simulink model "simple_router"  (R2015a)
settings: Solver=ode45  StartTime=0.0  StopTime=3000  FixedStep=1  RelTol=1e-3
undefined symbols (not defined in the file or in its folder): des, SELECT, T
libraries: simulink x16
(part 4 of 6)

== system simple_router/PE3/Create Generator Selection Variable ==
  function : TriggerPort  TriggerType=function-call
  Repeating Sequence Stair : simulink/Sources/Repeating Sequence Stair  OutValues=[0 1].'  tsamp=-1  OutMin=[]  OutMax=[]  OutDataTypeStr=float('double')  OutputDataTypeScalingMode=Specify via dialog  OutDataType=float('double')  ConRadixGroup=Best Precision: Vector-wise  OutScaling=2^-12
  Out1 : Outport
  wires:
  Repeating Sequence Stair/1 -> Out1/1

== system simple_router/PE4/Create Generator Selection Variable ==
  function : TriggerPort  TriggerType=function-call
  Repeating Sequence Stair : simulink/Sources/Repeating Sequence Stair  OutValues=[0 1].'  tsamp=-1  OutMin=[]  OutMax=[]  OutDataTypeStr=float('double')  OutputDataTypeScalingMode=Specify via dialog  OutDataType=float('double')  ConRadixGroup=Best Precision: Vector-wise  OutScaling=2^-12
  Out1 : Outport
  wires:
  Repeating Sequence Stair/1 -> Out1/1

== system simple_router/PE5/Create Generator Selection Variable ==
  function : TriggerPort  TriggerType=function-call
  Repeating Sequence Stair : simulink/Sources/Repeating Sequence Stair  OutValues=[0 1].'  tsamp=-1  OutMin=[]  OutMax=[]  OutDataTypeStr=float('double')  OutputDataTypeScalingMode=Specify via dialog  OutDataType=float('double')  ConRadixGroup=Best Precision: Vector-wise  OutScaling=2^-12
  Out1 : Outport
  wires:
  Repeating Sequence Stair/1 -> Out1/1

== system simple_router/PE6/Create Generator Selection Variable ==
  function : TriggerPort  TriggerType=function-call
  Repeating Sequence Stair : simulink/Sources/Repeating Sequence Stair  OutValues=[0 1].'  tsamp=-1  OutMin=[]  OutMax=[]  OutDataTypeStr=float('double')  OutputDataTypeScalingMode=Specify via dialog  OutDataType=float('double')  ConRadixGroup=Best Precision: Vector-wise  OutScaling=2^-12
  Out1 : Outport
  wires:
  Repeating Sequence Stair/1 -> Out1/1

== system simple_router/PE7/Create Generator Selection Variable ==
  function : TriggerPort  TriggerType=function-call
  Repeating Sequence Stair : simulink/Sources/Repeating Sequence Stair  OutValues=[0 1].'  tsamp=-1  OutMin=[]  OutMax=[]  OutDataTypeStr=float('double')  OutputDataTypeScalingMode=Specify via dialog  OutDataType=float('double')  ConRadixGroup=Best Precision: Vector-wise  OutScaling=2^-12
  Out1 : Outport
  wires:
  Repeating Sequence Stair/1 -> Out1/1

== system simple_router/PE8/Create Generator Selection Variable ==
  function : TriggerPort  TriggerType=function-call
  Repeating Sequence Stair : simulink/Sources/Repeating Sequence Stair  OutValues=[0 1].'  tsamp=-1  OutMin=[]  OutMax=[]  OutDataTypeStr=float('double')  OutputDataTypeScalingMode=Specify via dialog  OutDataType=float('double')  ConRadixGroup=Best Precision: Vector-wise  OutScaling=2^-12
  Out1 : Outport
  wires:
  Repeating Sequence Stair/1 -> Out1/1

== system simple_router/PE9/Create Generator Selection Variable ==
  function : TriggerPort  TriggerType=function-call
  Repeating Sequence Stair : simulink/Sources/Repeating Sequence Stair  OutValues=[0 1].'  tsamp=-1  OutMin=[]  OutMax=[]  OutDataTypeStr=float('double')  OutputDataTypeScalingMode=Specify via dialog  OutDataType=float('double')  ConRadixGroup=Best Precision: Vector-wise  OutScaling=2^-12
  Out1 : Outport
  wires:
  Repeating Sequence Stair/1 -> Out1/1

== system simple_router/Router00/Attribute Function ==
  MATLAB Function : MATLAB Function  TreatAsAtomicUnit=on
  __DMLF__EDE2FCE__ : EntityDepartureFunctionCallGenerator  TimingFunctionCallF1=Before entity departure  IsInsideAFB=on
  __DMLF__GA__ : GetAttribute  AttributeName=DST|ME  AttributeMissing=Error|Error  AttributeDefaultValue=1|1  AttributeTreatAsVector=1|1  AttributeSendTiming=Before entity departure|Before entity departure  EvaluatedDefaultAttributeValue={ [];[]}  IsInsideAFB=on
      settings: OutputPortMap=o1,o2
  __DMLF__SA__ : SetAttribute  AttributeName=RT  AttributeFrom=Signal port  EvaluatedAttributeValue={ []}  IsInsideAFB=on
  IN : PMIOPort  Port=1  Side=Left
  OUT : PMIOPort  Port=2  Side=Right
  wires:
  __DMLF__EDE2FCE__/1 -> MATLAB Function/Trigger
  __DMLF__GA__/1 -> MATLAB Function/1(DST)
  __DMLF__GA__/2 -> MATLAB Function/2(ME)
  MATLAB Function/1(out_RT) -> __DMLF__SA__/1
  connections:
  __DMLF__SA__/LConn1 -- __DMLF__EDE2FCE__/RConn1
  __DMLF__GA__/RConn1 -- __DMLF__EDE2FCE__/LConn1
  IN/RConn1 -- __DMLF__GA__/LConn1
  __DMLF__SA__/RConn1 -- OUT/RConn1

== system simple_router/Router00/Clocked FIFO1 ==
  Event-Based Random Number : EventBasedRandomNumber  Distribution=Gaussian (normal)  meanNorm=E  stdNorm=S
  FIFO Queue : FIFOQueue  Capacity=F  StatNumberInBlock=on
      settings: OutputPortMap=o1
  Release Gate : ReleaseGate  OpenGateUpon=Function call from port fcn
  Time-Based Function-Call Generator : TimeBasedFunctionCallGenerator  EventGenerationMode=Period from port  Period=T
  Input : PMIOPort  Port=1  Side=Left
  Output : PMIOPort  Port=2  Side=Right
  #n : Outport
  wires:
  Time-Based Function-Call Generator/1 -> Release Gate/1
  FIFO Queue/1 -> #n/1
  Event-Based Random Number/1 -> Time-Based Function-Call Generator/1
  connections:
  FIFO Queue/LConn1 -- Input/RConn1
  Release Gate/RConn1 -- Output/RConn1
  FIFO Queue/RConn1 -- Release Gate/LConn1

== system simple_router/Router00/Clocked FIFO2 ==
  Event-Based Random Number : EventBasedRandomNumber  Distribution=Gaussian (normal)  meanNorm=E  stdNorm=S
  FIFO Queue : FIFOQueue  Capacity=F  StatNumberInBlock=on
      settings: OutputPortMap=o1
  Release Gate : ReleaseGate  OpenGateUpon=Function call from port fcn
  Time-Based Function-Call Generator : TimeBasedFunctionCallGenerator  EventGenerationMode=Period from port  Period=T
  Input : PMIOPort  Port=1  Side=Left
  Output : PMIOPort  Port=2  Side=Right
  #n : Outport
  wires:
  Time-Based Function-Call Generator/1 -> Release Gate/1
  FIFO Queue/1 -> #n/1
  Event-Based Random Number/1 -> Time-Based Function-Call Generator/1
  connections:
  FIFO Queue/LConn1 -- Input/RConn1
  Release Gate/RConn1 -- Output/RConn1
  FIFO Queue/RConn1 -- Release Gate/LConn1

== system simple_router/Router00/Clocked FIFO3 ==
  Event-Based Random Number : EventBasedRandomNumber  Distribution=Gaussian (normal)  meanNorm=E  stdNorm=S
  FIFO Queue : FIFOQueue  Capacity=F  StatNumberInBlock=on
      settings: OutputPortMap=o1
  Release Gate : ReleaseGate  OpenGateUpon=Function call from port fcn
  Time-Based Function-Call Generator : TimeBasedFunctionCallGenerator  EventGenerationMode=Period from port  Period=T
  Input : PMIOPort  Port=1  Side=Left
  Output : PMIOPort  Port=2  Side=Right
  #n : Outport
  wires:
  Time-Based Function-Call Generator/1 -> Release Gate/1
  FIFO Queue/1 -> #n/1
  Event-Based Random Number/1 -> Time-Based Function-Call Generator/1
  connections:
  FIFO Queue/LConn1 -- Input/RConn1
  Release Gate/RConn1 -- Output/RConn1
  FIFO Queue/RConn1 -- Release Gate/LConn1

== system simple_router/Router00/Clocked FIFO4 ==
  Event-Based Random Number : EventBasedRandomNumber  Distribution=Gaussian (normal)  meanNorm=E  stdNorm=S
  FIFO Queue : FIFOQueue  Capacity=F  StatNumberInBlock=on
      settings: OutputPortMap=o1
  Release Gate : ReleaseGate  OpenGateUpon=Function call from port fcn
  Time-Based Function-Call Generator : TimeBasedFunctionCallGenerator  EventGenerationMode=Period from port  Period=T
  Input : PMIOPort  Port=1  Side=Left
  Output : PMIOPort  Port=2  Side=Right
  #n : Outport
  wires:
  Time-Based Function-Call Generator/1 -> Release Gate/1
  FIFO Queue/1 -> #n/1
  Event-Based Random Number/1 -> Time-Based Function-Call Generator/1
  connections:
  FIFO Queue/LConn1 -- Input/RConn1
  Release Gate/RConn1 -- Output/RConn1
  FIFO Queue/RConn1 -- Release Gate/LConn1

== system simple_router/Router00/Clocked FIFO5 ==
  Event-Based Random Number : EventBasedRandomNumber  Distribution=Gaussian (normal)  meanNorm=E  stdNorm=S
  FIFO Queue : FIFOQueue  Capacity=F  StatNumberInBlock=on
      settings: OutputPortMap=o1
  Release Gate : ReleaseGate  OpenGateUpon=Function call from port fcn
  Time-Based Function-Call Generator : TimeBasedFunctionCallGenerator  EventGenerationMode=Period from port  Period=T
  Input : PMIOPort  Port=1  Side=Left
  Output : PMIOPort  Port=2  Side=Right
  #n : Outport
  wires:
  Time-Based Function-Call Generator/1 -> Release Gate/1
  FIFO Queue/1 -> #n/1
  Event-Based Random Number/1 -> Time-Based Function-Call Generator/1
  connections:
  FIFO Queue/LConn1 -- Input/RConn1
  Release Gate/RConn1 -- Output/RConn1
  FIFO Queue/RConn1 -- Release Gate/LConn1

== system simple_router/Router01/Attribute Function ==
  MATLAB Function : MATLAB Function  TreatAsAtomicUnit=on
  __DMLF__EDE2FCE__ : EntityDepartureFunctionCallGenerator  TimingFunctionCallF1=Before entity departure  IsInsideAFB=on
  __DMLF__GA__ : GetAttribute  AttributeName=DST|ME  AttributeMissing=Error|Error  AttributeDefaultValue=1|1  AttributeTreatAsVector=1|1  AttributeSendTiming=Before entity departure|Before entity departure  EvaluatedDefaultAttributeValue={ [];[]}  IsInsideAFB=on
      settings: OutputPortMap=o1,o2
  __DMLF__SA__ : SetAttribute  AttributeName=RT  AttributeFrom=Signal port  EvaluatedAttributeValue={ []}  IsInsideAFB=on
  IN : PMIOPort  Port=1  Side=Left
  OUT : PMIOPort  Port=2  Side=Right
  wires:
  __DMLF__EDE2FCE__/1 -> MATLAB Function/Trigger
  __DMLF__GA__/1 -> MATLAB Function/1(DST)
  __DMLF__GA__/2 -> MATLAB Function/2(ME)
  MATLAB Function/1(out_RT) -> __DMLF__SA__/1
  connections:
  __DMLF__SA__/LConn1 -- __DMLF__EDE2FCE__/RConn1
  __DMLF__GA__/RConn1 -- __DMLF__EDE2FCE__/LConn1
  IN/RConn1 -- __DMLF__GA__/LConn1
  __DMLF__SA__/RConn1 -- OUT/RConn1

== system simple_router/Router01/Clocked FIFO1 ==
  Event-Based Random Number : EventBasedRandomNumber  Distribution=Gaussian (normal)  meanNorm=E  stdNorm=S
  FIFO Queue : FIFOQueue  Capacity=F  StatNumberInBlock=on
      settings: OutputPortMap=o1
  Release Gate : ReleaseGate  OpenGateUpon=Function call from port fcn
  Time-Based Function-Call Generator : TimeBasedFunctionCallGenerator  EventGenerationMode=Period from port  Period=T
  Input : PMIOPort  Port=1  Side=Left
  Output : PMIOPort  Port=2  Side=Right
  #n : Outport
  wires:
  Time-Based Function-Call Generator/1 -> Release Gate/1
  FIFO Queue/1 -> #n/1
  Event-Based Random Number/1 -> Time-Based Function-Call Generator/1
  connections:
  FIFO Queue/LConn1 -- Input/RConn1
  Release Gate/RConn1 -- Output/RConn1
  FIFO Queue/RConn1 -- Release Gate/LConn1

== system simple_router/Router01/Clocked FIFO2 ==
  Event-Based Random Number : EventBasedRandomNumber  Distribution=Gaussian (normal)  meanNorm=E  stdNorm=S
  FIFO Queue : FIFOQueue  Capacity=F  StatNumberInBlock=on
      settings: OutputPortMap=o1
  Release Gate : ReleaseGate  OpenGateUpon=Function call from port fcn
  Time-Based Function-Call Generator : TimeBasedFunctionCallGenerator  EventGenerationMode=Period from port  Period=T
  Input : PMIOPort  Port=1  Side=Left
  Output : PMIOPort  Port=2  Side=Right
  #n : Outport
  wires:
  Time-Based Function-Call Generator/1 -> Release Gate/1
  FIFO Queue/1 -> #n/1
  Event-Based Random Number/1 -> Time-Based Function-Call Generator/1
  connections:
  FIFO Queue/LConn1 -- Input/RConn1
  Release Gate/RConn1 -- Output/RConn1
  FIFO Queue/RConn1 -- Release Gate/LConn1

== system simple_router/Router01/Clocked FIFO3 ==
  Event-Based Random Number : EventBasedRandomNumber  Distribution=Gaussian (normal)  meanNorm=E  stdNorm=S
  FIFO Queue : FIFOQueue  Capacity=F  StatNumberInBlock=on
      settings: OutputPortMap=o1
  Release Gate : ReleaseGate  OpenGateUpon=Function call from port fcn
  Time-Based Function-Call Generator : TimeBasedFunctionCallGenerator  EventGenerationMode=Period from port  Period=T
  Input : PMIOPort  Port=1  Side=Left
  Output : PMIOPort  Port=2  Side=Right
  #n : Outport
  wires:
  Time-Based Function-Call Generator/1 -> Release Gate/1
  FIFO Queue/1 -> #n/1
  Event-Based Random Number/1 -> Time-Based Function-Call Generator/1
  connections:
  FIFO Queue/LConn1 -- Input/RConn1
  Release Gate/RConn1 -- Output/RConn1
  FIFO Queue/RConn1 -- Release Gate/LConn1

== system simple_router/Router01/Clocked FIFO4 ==
  Event-Based Random Number : EventBasedRandomNumber  Distribution=Gaussian (normal)  meanNorm=E  stdNorm=S
  FIFO Queue : FIFOQueue  Capacity=F  StatNumberInBlock=on
      settings: OutputPortMap=o1
  Release Gate : ReleaseGate  OpenGateUpon=Function call from port fcn
  Time-Based Function-Call Generator : TimeBasedFunctionCallGenerator  EventGenerationMode=Period from port  Period=T
  Input : PMIOPort  Port=1  Side=Left
  Output : PMIOPort  Port=2  Side=Right
  #n : Outport
  wires:
  Time-Based Function-Call Generator/1 -> Release Gate/1
  FIFO Queue/1 -> #n/1
  Event-Based Random Number/1 -> Time-Based Function-Call Generator/1
  connections:
  FIFO Queue/LConn1 -- Input/RConn1
  Release Gate/RConn1 -- Output/RConn1
  FIFO Queue/RConn1 -- Release Gate/LConn1

== system simple_router/Router01/Clocked FIFO5 ==
  Event-Based Random Number : EventBasedRandomNumber  Distribution=Gaussian (normal)  meanNorm=E  stdNorm=S
  FIFO Queue : FIFOQueue  Capacity=F  StatNumberInBlock=on
      settings: OutputPortMap=o1
  Release Gate : ReleaseGate  OpenGateUpon=Function call from port fcn
  Time-Based Function-Call Generator : TimeBasedFunctionCallGenerator  EventGenerationMode=Period from port  Period=T
  Input : PMIOPort  Port=1  Side=Left
  Output : PMIOPort  Port=2  Side=Right
  #n : Outport
  wires:
  Time-Based Function-Call Generator/1 -> Release Gate/1
  FIFO Queue/1 -> #n/1
  Event-Based Random Number/1 -> Time-Based Function-Call Generator/1
  connections:
  FIFO Queue/LConn1 -- Input/RConn1
  Release Gate/RConn1 -- Output/RConn1
  FIFO Queue/RConn1 -- Release Gate/LConn1

== system simple_router/Router02/Attribute Function ==
  MATLAB Function : MATLAB Function  TreatAsAtomicUnit=on
  __DMLF__EDE2FCE__ : EntityDepartureFunctionCallGenerator  TimingFunctionCallF1=Before entity departure  IsInsideAFB=on
  __DMLF__GA__ : GetAttribute  AttributeName=DST|ME  AttributeMissing=Error|Error  AttributeDefaultValue=1|1  AttributeTreatAsVector=1|1  AttributeSendTiming=Before entity departure|Before entity departure  EvaluatedDefaultAttributeValue={ [];[]}  IsInsideAFB=on
      settings: OutputPortMap=o1,o2
  __DMLF__SA__ : SetAttribute  AttributeName=RT  AttributeFrom=Signal port  EvaluatedAttributeValue={ []}  IsInsideAFB=on
  IN : PMIOPort  Port=1  Side=Left
  OUT : PMIOPort  Port=2  Side=Right
  wires:
  __DMLF__EDE2FCE__/1 -> MATLAB Function/Trigger
  __DMLF__GA__/1 -> MATLAB Function/1(DST)
  __DMLF__GA__/2 -> MATLAB Function/2(ME)
  MATLAB Function/1(out_RT) -> __DMLF__SA__/1
  connections:
  __DMLF__SA__/LConn1 -- __DMLF__EDE2FCE__/RConn1
  __DMLF__GA__/RConn1 -- __DMLF__EDE2FCE__/LConn1
  IN/RConn1 -- __DMLF__GA__/LConn1
  __DMLF__SA__/RConn1 -- OUT/RConn1

== system simple_router/Router02/Clocked FIFO1 ==
  Event-Based Random Number : EventBasedRandomNumber  Distribution=Gaussian (normal)  meanNorm=E  stdNorm=S
  FIFO Queue : FIFOQueue  Capacity=F  StatNumberInBlock=on
      settings: OutputPortMap=o1
  Release Gate : ReleaseGate  OpenGateUpon=Function call from port fcn
  Time-Based Function-Call Generator : TimeBasedFunctionCallGenerator  EventGenerationMode=Period from port  Period=T
  Input : PMIOPort  Port=1  Side=Left
  Output : PMIOPort  Port=2  Side=Right
  #n : Outport
  wires:
  Time-Based Function-Call Generator/1 -> Release Gate/1
  FIFO Queue/1 -> #n/1
  Event-Based Random Number/1 -> Time-Based Function-Call Generator/1
  connections:
  FIFO Queue/LConn1 -- Input/RConn1
  Release Gate/RConn1 -- Output/RConn1
  FIFO Queue/RConn1 -- Release Gate/LConn1

== system simple_router/Router02/Clocked FIFO2 ==
  Event-Based Random Number : EventBasedRandomNumber  Distribution=Gaussian (normal)  meanNorm=E  stdNorm=S
  FIFO Queue : FIFOQueue  Capacity=F  StatNumberInBlock=on
      settings: OutputPortMap=o1
  Release Gate : ReleaseGate  OpenGateUpon=Function call from port fcn
  Time-Based Function-Call Generator : TimeBasedFunctionCallGenerator  EventGenerationMode=Period from port  Period=T
  Input : PMIOPort  Port=1  Side=Left
  Output : PMIOPort  Port=2  Side=Right
  #n : Outport
  wires:
  Time-Based Function-Call Generator/1 -> Release Gate/1
  FIFO Queue/1 -> #n/1
  Event-Based Random Number/1 -> Time-Based Function-Call Generator/1
  connections:
  FIFO Queue/LConn1 -- Input/RConn1
  Release Gate/RConn1 -- Output/RConn1
  FIFO Queue/RConn1 -- Release Gate/LConn1

== system simple_router/Router02/Clocked FIFO3 ==
  Event-Based Random Number : EventBasedRandomNumber  Distribution=Gaussian (normal)  meanNorm=E  stdNorm=S
  FIFO Queue : FIFOQueue  Capacity=F  StatNumberInBlock=on
      settings: OutputPortMap=o1
  Release Gate : ReleaseGate  OpenGateUpon=Function call from port fcn
  Time-Based Function-Call Generator : TimeBasedFunctionCallGenerator  EventGenerationMode=Period from port  Period=T
  Input : PMIOPort  Port=1  Side=Left
  Output : PMIOPort  Port=2  Side=Right
  #n : Outport
  wires:
  Time-Based Function-Call Generator/1 -> Release Gate/1
  FIFO Queue/1 -> #n/1
  Event-Based Random Number/1 -> Time-Based Function-Call Generator/1
  connections:
  FIFO Queue/LConn1 -- Input/RConn1
  Release Gate/RConn1 -- Output/RConn1
  FIFO Queue/RConn1 -- Release Gate/LConn1

== system simple_router/Router02/Clocked FIFO4 ==
  Event-Based Random Number : EventBasedRandomNumber  Distribution=Gaussian (normal)  meanNorm=E  stdNorm=S
  FIFO Queue : FIFOQueue  Capacity=F  StatNumberInBlock=on
      settings: OutputPortMap=o1
  Release Gate : ReleaseGate  OpenGateUpon=Function call from port fcn
  Time-Based Function-Call Generator : TimeBasedFunctionCallGenerator  EventGenerationMode=Period from port  Period=T
  Input : PMIOPort  Port=1  Side=Left
  Output : PMIOPort  Port=2  Side=Right
  #n : Outport
  wires:
  Time-Based Function-Call Generator/1 -> Release Gate/1
  FIFO Queue/1 -> #n/1
  Event-Based Random Number/1 -> Time-Based Function-Call Generator/1
  connections:
  FIFO Queue/LConn1 -- Input/RConn1
  Release Gate/RConn1 -- Output/RConn1
  FIFO Queue/RConn1 -- Release Gate/LConn1

== system simple_router/Router02/Clocked FIFO5 ==
  Event-Based Random Number : EventBasedRandomNumber  Distribution=Gaussian (normal)  meanNorm=E  stdNorm=S
  FIFO Queue : FIFOQueue  Capacity=F  StatNumberInBlock=on
      settings: OutputPortMap=o1
  Release Gate : ReleaseGate  OpenGateUpon=Function call from port fcn
  Time-Based Function-Call Generator : TimeBasedFunctionCallGenerator  EventGenerationMode=Period from port  Period=T
  Input : PMIOPort  Port=1  Side=Left
  Output : PMIOPort  Port=2  Side=Right
  #n : Outport
  wires:
  Time-Based Function-Call Generator/1 -> Release Gate/1
  FIFO Queue/1 -> #n/1
  Event-Based Random Number/1 -> Time-Based Function-Call Generator/1
  connections:
  FIFO Queue/LConn1 -- Input/RConn1
  Release Gate/RConn1 -- Output/RConn1
  FIFO Queue/RConn1 -- Release Gate/LConn1

== system simple_router/Router03/Attribute Function ==
  MATLAB Function : MATLAB Function  TreatAsAtomicUnit=on
  __DMLF__EDE2FCE__ : EntityDepartureFunctionCallGenerator  TimingFunctionCallF1=Before entity departure  IsInsideAFB=on
  __DMLF__GA__ : GetAttribute  AttributeName=DST|ME  AttributeMissing=Error|Error  AttributeDefaultValue=1|1  AttributeTreatAsVector=1|1  AttributeSendTiming=Before entity departure|Before entity departure  EvaluatedDefaultAttributeValue={ [];[]}  IsInsideAFB=on
      settings: OutputPortMap=o1,o2
  __DMLF__SA__ : SetAttribute  AttributeName=RT  AttributeFrom=Signal port  EvaluatedAttributeValue={ []}  IsInsideAFB=on
  IN : PMIOPort  Port=1  Side=Left
  OUT : PMIOPort  Port=2  Side=Right
  wires:
  __DMLF__EDE2FCE__/1 -> MATLAB Function/Trigger
  __DMLF__GA__/1 -> MATLAB Function/1(DST)
  __DMLF__GA__/2 -> MATLAB Function/2(ME)
  MATLAB Function/1(out_RT) -> __DMLF__SA__/1
  connections:
  __DMLF__SA__/LConn1 -- __DMLF__EDE2FCE__/RConn1
  __DMLF__GA__/RConn1 -- __DMLF__EDE2FCE__/LConn1
  IN/RConn1 -- __DMLF__GA__/LConn1
  __DMLF__SA__/RConn1 -- OUT/RConn1

== system simple_router/Router03/Clocked FIFO1 ==
  Event-Based Random Number : EventBasedRandomNumber  Distribution=Gaussian (normal)  meanNorm=E  stdNorm=S
  FIFO Queue : FIFOQueue  Capacity=F  StatNumberInBlock=on
      settings: OutputPortMap=o1
  Release Gate : ReleaseGate  OpenGateUpon=Function call from port fcn
  Time-Based Function-Call Generator : TimeBasedFunctionCallGenerator  EventGenerationMode=Period from port  Period=T
  Input : PMIOPort  Port=1  Side=Left
  Output : PMIOPort  Port=2  Side=Right
  #n : Outport
  wires:
  Time-Based Function-Call Generator/1 -> Release Gate/1
  FIFO Queue/1 -> #n/1
  Event-Based Random Number/1 -> Time-Based Function-Call Generator/1
  connections:
  FIFO Queue/LConn1 -- Input/RConn1
  Release Gate/RConn1 -- Output/RConn1
  FIFO Queue/RConn1 -- Release Gate/LConn1

== system simple_router/Router03/Clocked FIFO2 ==
  Event-Based Random Number : EventBasedRandomNumber  Distribution=Gaussian (normal)  meanNorm=E  stdNorm=S
  FIFO Queue : FIFOQueue  Capacity=F  StatNumberInBlock=on
      settings: OutputPortMap=o1
  Release Gate : ReleaseGate  OpenGateUpon=Function call from port fcn
  Time-Based Function-Call Generator : TimeBasedFunctionCallGenerator  EventGenerationMode=Period from port  Period=T
  Input : PMIOPort  Port=1  Side=Left
  Output : PMIOPort  Port=2  Side=Right
  #n : Outport
  wires:
  Time-Based Function-Call Generator/1 -> Release Gate/1
  FIFO Queue/1 -> #n/1
  Event-Based Random Number/1 -> Time-Based Function-Call Generator/1
  connections:
  FIFO Queue/LConn1 -- Input/RConn1
  Release Gate/RConn1 -- Output/RConn1
  FIFO Queue/RConn1 -- Release Gate/LConn1

== system simple_router/Router03/Clocked FIFO3 ==
  Event-Based Random Number : EventBasedRandomNumber  Distribution=Gaussian (normal)  meanNorm=E  stdNorm=S
  FIFO Queue : FIFOQueue  Capacity=F  StatNumberInBlock=on
      settings: OutputPortMap=o1
  Release Gate : ReleaseGate  OpenGateUpon=Function call from port fcn
  Time-Based Function-Call Generator : TimeBasedFunctionCallGenerator  EventGenerationMode=Period from port  Period=T
  Input : PMIOPort  Port=1  Side=Left
  Output : PMIOPort  Port=2  Side=Right
  #n : Outport
  wires:
  Time-Based Function-Call Generator/1 -> Release Gate/1
  FIFO Queue/1 -> #n/1
  Event-Based Random Number/1 -> Time-Based Function-Call Generator/1
  connections:
  FIFO Queue/LConn1 -- Input/RConn1
  Release Gate/RConn1 -- Output/RConn1
  FIFO Queue/RConn1 -- Release Gate/LConn1

== system simple_router/Router03/Clocked FIFO4 ==
  Event-Based Random Number : EventBasedRandomNumber  Distribution=Gaussian (normal)  meanNorm=E  stdNorm=S
  FIFO Queue : FIFOQueue  Capacity=F  StatNumberInBlock=on
      settings: OutputPortMap=o1
  Release Gate : ReleaseGate  OpenGateUpon=Function call from port fcn
  Time-Based Function-Call Generator : TimeBasedFunctionCallGenerator  EventGenerationMode=Period from port  Period=T
  Input : PMIOPort  Port=1  Side=Left
  Output : PMIOPort  Port=2  Side=Right
  #n : Outport
  wires:
  Time-Based Function-Call Generator/1 -> Release Gate/1
  FIFO Queue/1 -> #n/1
  Event-Based Random Number/1 -> Time-Based Function-Call Generator/1
  connections:
  FIFO Queue/LConn1 -- Input/RConn1
  Release Gate/RConn1 -- Output/RConn1
  FIFO Queue/RConn1 -- Release Gate/LConn1

== system simple_router/Router03/Clocked FIFO5 ==
  Event-Based Random Number : EventBasedRandomNumber  Distribution=Gaussian (normal)  meanNorm=E  stdNorm=S
  FIFO Queue : FIFOQueue  Capacity=F  StatNumberInBlock=on
      settings: OutputPortMap=o1
  Release Gate : ReleaseGate  OpenGateUpon=Function call from port fcn
  Time-Based Function-Call Generator : TimeBasedFunctionCallGenerator  EventGenerationMode=Period from port  Period=T
  Input : PMIOPort  Port=1  Side=Left
  Output : PMIOPort  Port=2  Side=Right
  #n : Outport
  wires:
  Time-Based Function-Call Generator/1 -> Release Gate/1
  FIFO Queue/1 -> #n/1
  Event-Based Random Number/1 -> Time-Based Function-Call Generator/1
  connections:
  FIFO Queue/LConn1 -- Input/RConn1
  Release Gate/RConn1 -- Output/RConn1
  FIFO Queue/RConn1 -- Release Gate/LConn1

== system simple_router/Router09/Attribute Function ==
  MATLAB Function : MATLAB Function  TreatAsAtomicUnit=on
  __DMLF__EDE2FCE__ : EntityDepartureFunctionCallGenerator  TimingFunctionCallF1=Before entity departure  IsInsideAFB=on
  __DMLF__GA__ : GetAttribute  AttributeName=DST|ME  AttributeMissing=Error|Error  AttributeDefaultValue=1|1  AttributeTreatAsVector=1|1  AttributeSendTiming=Before entity departure|Before entity departure  EvaluatedDefaultAttributeValue={ [];[]}  IsInsideAFB=on
      settings: OutputPortMap=o1,o2
  __DMLF__SA__ : SetAttribute  AttributeName=RT  AttributeFrom=Signal port  EvaluatedAttributeValue={ []}  IsInsideAFB=on
  IN : PMIOPort  Port=1  Side=Left
  OUT : PMIOPort  Port=2  Side=Right
  wires:
  __DMLF__EDE2FCE__/1 -> MATLAB Function/Trigger
  __DMLF__GA__/1 -> MATLAB Function/1(DST)
  __DMLF__GA__/2 -> MATLAB Function/2(ME)
  MATLAB Function/1(out_RT) -> __DMLF__SA__/1
  connections:
  __DMLF__SA__/LConn1 -- __DMLF__EDE2FCE__/RConn1
  __DMLF__GA__/RConn1 -- __DMLF__EDE2FCE__/LConn1
  IN/RConn1 -- __DMLF__GA__/LConn1
  __DMLF__SA__/RConn1 -- OUT/RConn1

== system simple_router/Router09/Clocked FIFO1 ==
  Event-Based Random Number : EventBasedRandomNumber  Distribution=Gaussian (normal)  meanNorm=E  stdNorm=S
  FIFO Queue : FIFOQueue  Capacity=F  StatNumberInBlock=on
      settings: OutputPortMap=o1
  Release Gate : ReleaseGate  OpenGateUpon=Function call from port fcn
  Time-Based Function-Call Generator : TimeBasedFunctionCallGenerator  EventGenerationMode=Period from port  Period=T
  Input : PMIOPort  Port=1  Side=Left
  Output : PMIOPort  Port=2  Side=Right
  #n : Outport
  wires:
  Time-Based Function-Call Generator/1 -> Release Gate/1
  FIFO Queue/1 -> #n/1
  Event-Based Random Number/1 -> Time-Based Function-Call Generator/1
  connections:
  FIFO Queue/LConn1 -- Input/RConn1
  Release Gate/RConn1 -- Output/RConn1
  FIFO Queue/RConn1 -- Release Gate/LConn1

== system simple_router/Router09/Clocked FIFO2 ==
  Event-Based Random Number : EventBasedRandomNumber  Distribution=Gaussian (normal)  meanNorm=E  stdNorm=S
  FIFO Queue : FIFOQueue  Capacity=F  StatNumberInBlock=on
      settings: OutputPortMap=o1
  Release Gate : ReleaseGate  OpenGateUpon=Function call from port fcn
  Time-Based Function-Call Generator : TimeBasedFunctionCallGenerator  EventGenerationMode=Period from port  Period=T
  Input : PMIOPort  Port=1  Side=Left
  Output : PMIOPort  Port=2  Side=Right
  #n : Outport
  wires:
  Time-Based Function-Call Generator/1 -> Release Gate/1
  FIFO Queue/1 -> #n/1
  Event-Based Random Number/1 -> Time-Based Function-Call Generator/1
  connections:
  FIFO Queue/LConn1 -- Input/RConn1
  Release Gate/RConn1 -- Output/RConn1
  FIFO Queue/RConn1 -- Release Gate/LConn1

== system simple_router/Router09/Clocked FIFO3 ==
  Event-Based Random Number : EventBasedRandomNumber  Distribution=Gaussian (normal)  meanNorm=E  stdNorm=S
  FIFO Queue : FIFOQueue  Capacity=F  StatNumberInBlock=on
      settings: OutputPortMap=o1
  Release Gate : ReleaseGate  OpenGateUpon=Function call from port fcn
  Time-Based Function-Call Generator : TimeBasedFunctionCallGenerator  EventGenerationMode=Period from port  Period=T
  Input : PMIOPort  Port=1  Side=Left
  Output : PMIOPort  Port=2  Side=Right
  #n : Outport
  wires:
  Time-Based Function-Call Generator/1 -> Release Gate/1
  FIFO Queue/1 -> #n/1
  Event-Based Random Number/1 -> Time-Based Function-Call Generator/1
  connections:
  FIFO Queue/LConn1 -- Input/RConn1
  Release Gate/RConn1 -- Output/RConn1
  FIFO Queue/RConn1 -- Release Gate/LConn1

== system simple_router/Router09/Clocked FIFO4 ==
  Event-Based Random Number : EventBasedRandomNumber  Distribution=Gaussian (normal)  meanNorm=E  stdNorm=S
  FIFO Queue : FIFOQueue  Capacity=F  StatNumberInBlock=on
      settings: OutputPortMap=o1
  Release Gate : ReleaseGate  OpenGateUpon=Function call from port fcn
  Time-Based Function-Call Generator : TimeBasedFunctionCallGenerator  EventGenerationMode=Period from port  Period=T
  Input : PMIOPort  Port=1  Side=Left
  Output : PMIOPort  Port=2  Side=Right
  #n : Outport
  wires:
  Time-Based Function-Call Generator/1 -> Release Gate/1
  FIFO Queue/1 -> #n/1
  Event-Based Random Number/1 -> Time-Based Function-Call Generator/1
  connections:
  FIFO Queue/LConn1 -- Input/RConn1
  Release Gate/RConn1 -- Output/RConn1
  FIFO Queue/RConn1 -- Release Gate/LConn1

== system simple_router/Router09/Clocked FIFO5 ==
  Event-Based Random Number : EventBasedRandomNumber  Distribution=Gaussian (normal)  meanNorm=E  stdNorm=S
  FIFO Queue : FIFOQueue  Capacity=F  StatNumberInBlock=on
      settings: OutputPortMap=o1
  Release Gate : ReleaseGate  OpenGateUpon=Function call from port fcn
  Time-Based Function-Call Generator : TimeBasedFunctionCallGenerator  EventGenerationMode=Period from port  Period=T
  Input : PMIOPort  Port=1  Side=Left
  Output : PMIOPort  Port=2  Side=Right
  #n : Outport
  wires:
  Time-Based Function-Call Generator/1 -> Release Gate/1
  FIFO Queue/1 -> #n/1
  Event-Based Random Number/1 -> Time-Based Function-Call Generator/1
  connections:
  FIFO Queue/LConn1 -- Input/RConn1
  Release Gate/RConn1 -- Output/RConn1
  FIFO Queue/RConn1 -- Release Gate/LConn1

== system simple_router/Router10/Attribute Function ==
  MATLAB Function : MATLAB Function  TreatAsAtomicUnit=on
  __DMLF__EDE2FCE__ : EntityDepartureFunctionCallGenerator  TimingFunctionCallF1=Before entity departure  IsInsideAFB=on
  __DMLF__GA__ : GetAttribute  AttributeName=DST|ME  AttributeMissing=Error|Error  AttributeDefaultValue=1|1  AttributeTreatAsVector=1|1  AttributeSendTiming=Before entity departure|Before entity departure  EvaluatedDefaultAttributeValue={ [];[]}  IsInsideAFB=on
      settings: OutputPortMap=o1,o2
  __DMLF__SA__ : SetAttribute  AttributeName=RT  AttributeFrom=Signal port  EvaluatedAttributeValue={ []}  IsInsideAFB=on
  IN : PMIOPort  Port=1  Side=Left
  OUT : PMIOPort  Port=2  Side=Right
  wires:
  __DMLF__EDE2FCE__/1 -> MATLAB Function/Trigger
  __DMLF__GA__/1 -> MATLAB Function/1(DST)
  __DMLF__GA__/2 -> MATLAB Function/2(ME)
  MATLAB Function/1(out_RT) -> __DMLF__SA__/1
  connections:
  __DMLF__SA__/LConn1 -- __DMLF__EDE2FCE__/RConn1
  __DMLF__GA__/RConn1 -- __DMLF__EDE2FCE__/LConn1
  IN/RConn1 -- __DMLF__GA__/LConn1
  __DMLF__SA__/RConn1 -- OUT/RConn1

== system simple_router/Router10/Clocked FIFO1 ==
  Event-Based Random Number : EventBasedRandomNumber  Distribution=Gaussian (normal)  meanNorm=E  stdNorm=S
  FIFO Queue : FIFOQueue  Capacity=F  StatNumberInBlock=on
      settings: OutputPortMap=o1
  Release Gate : ReleaseGate  OpenGateUpon=Function call from port fcn
  Time-Based Function-Call Generator : TimeBasedFunctionCallGenerator  EventGenerationMode=Period from port  Period=T
  Input : PMIOPort  Port=1  Side=Left
  Output : PMIOPort  Port=2  Side=Right
  #n : Outport
  wires:
  Time-Based Function-Call Generator/1 -> Release Gate/1
  FIFO Queue/1 -> #n/1
  Event-Based Random Number/1 -> Time-Based Function-Call Generator/1
  connections:
  FIFO Queue/LConn1 -- Input/RConn1
  Release Gate/RConn1 -- Output/RConn1
  FIFO Queue/RConn1 -- Release Gate/LConn1

== system simple_router/Router10/Clocked FIFO2 ==
  Event-Based Random Number : EventBasedRandomNumber  Distribution=Gaussian (normal)  meanNorm=E  stdNorm=S
  FIFO Queue : FIFOQueue  Capacity=F  StatNumberInBlock=on
      settings: OutputPortMap=o1
  Release Gate : ReleaseGate  OpenGateUpon=Function call from port fcn
  Time-Based Function-Call Generator : TimeBasedFunctionCallGenerator  EventGenerationMode=Period from port  Period=T
  Input : PMIOPort  Port=1  Side=Left
  Output : PMIOPort  Port=2  Side=Right
  #n : Outport
  wires:
  Time-Based Function-Call Generator/1 -> Release Gate/1
  FIFO Queue/1 -> #n/1
  Event-Based Random Number/1 -> Time-Based Function-Call Generator/1
  connections:
  FIFO Queue/LConn1 -- Input/RConn1
  Release Gate/RConn1 -- Output/RConn1
  FIFO Queue/RConn1 -- Release Gate/LConn1

== system simple_router/Router10/Clocked FIFO3 ==
  Event-Based Random Number : EventBasedRandomNumber  Distribution=Gaussian (normal)  meanNorm=E  stdNorm=S
  FIFO Queue : FIFOQueue  Capacity=F  StatNumberInBlock=on
      settings: OutputPortMap=o1
  Release Gate : ReleaseGate  OpenGateUpon=Function call from port fcn
  Time-Based Function-Call Generator : TimeBasedFunctionCallGenerator  EventGenerationMode=Period from port  Period=T
  Input : PMIOPort  Port=1  Side=Left
  Output : PMIOPort  Port=2  Side=Right
  #n : Outport
  wires:
  Time-Based Function-Call Generator/1 -> Release Gate/1
  FIFO Queue/1 -> #n/1
  Event-Based Random Number/1 -> Time-Based Function-Call Generator/1
  connections:
  FIFO Queue/LConn1 -- Input/RConn1
  Release Gate/RConn1 -- Output/RConn1
  FIFO Queue/RConn1 -- Release Gate/LConn1

== system simple_router/Router10/Clocked FIFO4 ==
  Event-Based Random Number : EventBasedRandomNumber  Distribution=Gaussian (normal)  meanNorm=E  stdNorm=S
  FIFO Queue : FIFOQueue  Capacity=F  StatNumberInBlock=on
      settings: OutputPortMap=o1
  Release Gate : ReleaseGate  OpenGateUpon=Function call from port fcn
  Time-Based Function-Call Generator : TimeBasedFunctionCallGenerator  EventGenerationMode=Period from port  Period=T
  Input : PMIOPort  Port=1  Side=Left
  Output : PMIOPort  Port=2  Side=Right
  #n : Outport
  wires:
  Time-Based Function-Call Generator/1 -> Release Gate/1
  FIFO Queue/1 -> #n/1
  Event-Based Random Number/1 -> Time-Based Function-Call Generator/1
  connections:
  FIFO Queue/LConn1 -- Input/RConn1
  Release Gate/RConn1 -- Output/RConn1
  FIFO Queue/RConn1 -- Release Gate/LConn1

== system simple_router/Router10/Clocked FIFO5 ==
  Event-Based Random Number : EventBasedRandomNumber  Distribution=Gaussian (normal)  meanNorm=E  stdNorm=S
  FIFO Queue : FIFOQueue  Capacity=F  StatNumberInBlock=on
      settings: OutputPortMap=o1
  Release Gate : ReleaseGate  OpenGateUpon=Function call from port fcn
  Time-Based Function-Call Generator : TimeBasedFunctionCallGenerator  EventGenerationMode=Period from port  Period=T
  Input : PMIOPort  Port=1  Side=Left
  Output : PMIOPort  Port=2  Side=Right
  #n : Outport
  wires:
  Time-Based Function-Call Generator/1 -> Release Gate/1
  FIFO Queue/1 -> #n/1
  Event-Based Random Number/1 -> Time-Based Function-Call Generator/1
  connections:
  FIFO Queue/LConn1 -- Input/RConn1
  Release Gate/RConn1 -- Output/RConn1
  FIFO Queue/RConn1 -- Release Gate/LConn1

== system simple_router/Router11/Attribute Function ==
  MATLAB Function : MATLAB Function  TreatAsAtomicUnit=on
  __DMLF__EDE2FCE__ : EntityDepartureFunctionCallGenerator  TimingFunctionCallF1=Before entity departure  IsInsideAFB=on
  __DMLF__GA__ : GetAttribute  AttributeName=DST|ME  AttributeMissing=Error|Error  AttributeDefaultValue=1|1  AttributeTreatAsVector=1|1  AttributeSendTiming=Before entity departure|Before entity departure  EvaluatedDefaultAttributeValue={ [];[]}  IsInsideAFB=on
      settings: OutputPortMap=o1,o2
  __DMLF__SA__ : SetAttribute  AttributeName=RT  AttributeFrom=Signal port  EvaluatedAttributeValue={ []}  IsInsideAFB=on
  IN : PMIOPort  Port=1  Side=Left
  OUT : PMIOPort  Port=2  Side=Right
  wires:
  __DMLF__EDE2FCE__/1 -> MATLAB Function/Trigger
  __DMLF__GA__/1 -> MATLAB Function/1(DST)
  __DMLF__GA__/2 -> MATLAB Function/2(ME)
  MATLAB Function/1(out_RT) -> __DMLF__SA__/1
  connections:
  __DMLF__SA__/LConn1 -- __DMLF__EDE2FCE__/RConn1
  __DMLF__GA__/RConn1 -- __DMLF__EDE2FCE__/LConn1
  IN/RConn1 -- __DMLF__GA__/LConn1
  __DMLF__SA__/RConn1 -- OUT/RConn1

== system simple_router/Router11/Clocked FIFO1 ==
  Event-Based Random Number : EventBasedRandomNumber  Distribution=Gaussian (normal)  meanNorm=E  stdNorm=S
  FIFO Queue : FIFOQueue  Capacity=F  StatNumberInBlock=on
      settings: OutputPortMap=o1
  Release Gate : ReleaseGate  OpenGateUpon=Function call from port fcn
  Time-Based Function-Call Generator : TimeBasedFunctionCallGenerator  EventGenerationMode=Period from port  Period=T
  Input : PMIOPort  Port=1  Side=Left
  Output : PMIOPort  Port=2  Side=Right
  #n : Outport
  wires:
  Time-Based Function-Call Generator/1 -> Release Gate/1
  FIFO Queue/1 -> #n/1
  Event-Based Random Number/1 -> Time-Based Function-Call Generator/1
  connections:
  FIFO Queue/LConn1 -- Input/RConn1
  Release Gate/RConn1 -- Output/RConn1
  FIFO Queue/RConn1 -- Release Gate/LConn1

== system simple_router/Router11/Clocked FIFO2 ==
  Event-Based Random Number : EventBasedRandomNumber  Distribution=Gaussian (normal)  meanNorm=E  stdNorm=S
  FIFO Queue : FIFOQueue  Capacity=F  StatNumberInBlock=on
      settings: OutputPortMap=o1
  Release Gate : ReleaseGate  OpenGateUpon=Function call from port fcn
  Time-Based Function-Call Generator : TimeBasedFunctionCallGenerator  EventGenerationMode=Period from port  Period=T
  Input : PMIOPort  Port=1  Side=Left
  Output : PMIOPort  Port=2  Side=Right
  #n : Outport
  wires:
  Time-Based Function-Call Generator/1 -> Release Gate/1
  FIFO Queue/1 -> #n/1
  Event-Based Random Number/1 -> Time-Based Function-Call Generator/1
  connections:
  FIFO Queue/LConn1 -- Input/RConn1
  Release Gate/RConn1 -- Output/RConn1
  FIFO Queue/RConn1 -- Release Gate/LConn1

== system simple_router/Router11/Clocked FIFO3 ==
  Event-Based Random Number : EventBasedRandomNumber  Distribution=Gaussian (normal)  meanNorm=E  stdNorm=S
  FIFO Queue : FIFOQueue  Capacity=F  StatNumberInBlock=on
      settings: OutputPortMap=o1
  Release Gate : ReleaseGate  OpenGateUpon=Function call from port fcn
  Time-Based Function-Call Generator : TimeBasedFunctionCallGenerator  EventGenerationMode=Period from port  Period=T
  Input : PMIOPort  Port=1  Side=Left
  Output : PMIOPort  Port=2  Side=Right
  #n : Outport
  wires:
  Time-Based Function-Call Generator/1 -> Release Gate/1
  FIFO Queue/1 -> #n/1
  Event-Based Random Number/1 -> Time-Based Function-Call Generator/1
  connections:
  FIFO Queue/LConn1 -- Input/RConn1
  Release Gate/RConn1 -- Output/RConn1
  FIFO Queue/RConn1 -- Release Gate/LConn1

== system simple_router/Router11/Clocked FIFO4 ==
  Event-Based Random Number : EventBasedRandomNumber  Distribution=Gaussian (normal)  meanNorm=E  stdNorm=S
  FIFO Queue : FIFOQueue  Capacity=F  StatNumberInBlock=on
      settings: OutputPortMap=o1
  Release Gate : ReleaseGate  OpenGateUpon=Function call from port fcn
  Time-Based Function-Call Generator : TimeBasedFunctionCallGenerator  EventGenerationMode=Period from port  Period=T
  Input : PMIOPort  Port=1  Side=Left
  Output : PMIOPort  Port=2  Side=Right
  #n : Outport
  wires:
  Time-Based Function-Call Generator/1 -> Release Gate/1
  FIFO Queue/1 -> #n/1
  Event-Based Random Number/1 -> Time-Based Function-Call Generator/1
  connections:
  FIFO Queue/LConn1 -- Input/RConn1
  Release Gate/RConn1 -- Output/RConn1
  FIFO Queue/RConn1 -- Release Gate/LConn1

== system simple_router/Router11/Clocked FIFO5 ==
  Event-Based Random Number : EventBasedRandomNumber  Distribution=Gaussian (normal)  meanNorm=E  stdNorm=S
  FIFO Queue : FIFOQueue  Capacity=F  StatNumberInBlock=on
      settings: OutputPortMap=o1
  Release Gate : ReleaseGate  OpenGateUpon=Function call from port fcn
  Time-Based Function-Call Generator : TimeBasedFunctionCallGenerator  EventGenerationMode=Period from port  Period=T
  Input : PMIOPort  Port=1  Side=Left
  Output : PMIOPort  Port=2  Side=Right
  #n : Outport
  wires:
  Time-Based Function-Call Generator/1 -> Release Gate/1
  FIFO Queue/1 -> #n/1
  Event-Based Random Number/1 -> Time-Based Function-Call Generator/1
  connections:
  FIFO Queue/LConn1 -- Input/RConn1
  Release Gate/RConn1 -- Output/RConn1
  FIFO Queue/RConn1 -- Release Gate/LConn1

== system simple_router/Router12/Attribute Function ==
  MATLAB Function : MATLAB Function  TreatAsAtomicUnit=on
  __DMLF__EDE2FCE__ : EntityDepartureFunctionCallGenerator  TimingFunctionCallF1=Before entity departure  IsInsideAFB=on
  __DMLF__GA__ : GetAttribute  AttributeName=DST|ME  AttributeMissing=Error|Error  AttributeDefaultValue=1|1  AttributeTreatAsVector=1|1  AttributeSendTiming=Before entity departure|Before entity departure  EvaluatedDefaultAttributeValue={ [];[]}  IsInsideAFB=on
      settings: OutputPortMap=o1,o2
  __DMLF__SA__ : SetAttribute  AttributeName=RT  AttributeFrom=Signal port  EvaluatedAttributeValue={ []}  IsInsideAFB=on
  IN : PMIOPort  Port=1  Side=Left
  OUT : PMIOPort  Port=2  Side=Right
  wires:
  __DMLF__EDE2FCE__/1 -> MATLAB Function/Trigger
  __DMLF__GA__/1 -> MATLAB Function/1(DST)
  __DMLF__GA__/2 -> MATLAB Function/2(ME)
  MATLAB Function/1(out_RT) -> __DMLF__SA__/1
  connections:
  __DMLF__SA__/LConn1 -- __DMLF__EDE2FCE__/RConn1
  __DMLF__GA__/RConn1 -- __DMLF__EDE2FCE__/LConn1
  IN/RConn1 -- __DMLF__GA__/LConn1
  __DMLF__SA__/RConn1 -- OUT/RConn1

== system simple_router/Router12/Clocked FIFO1 ==
  Event-Based Random Number : EventBasedRandomNumber  Distribution=Gaussian (normal)  meanNorm=E  stdNorm=S
  FIFO Queue : FIFOQueue  Capacity=F  StatNumberInBlock=on
      settings: OutputPortMap=o1
  Release Gate : ReleaseGate  OpenGateUpon=Function call from port fcn
  Time-Based Function-Call Generator : TimeBasedFunctionCallGenerator  EventGenerationMode=Period from port  Period=T
  Input : PMIOPort  Port=1  Side=Left
  Output : PMIOPort  Port=2  Side=Right
  #n : Outport
  wires:
  Time-Based Function-Call Generator/1 -> Release Gate/1
  FIFO Queue/1 -> #n/1
  Event-Based Random Number/1 -> Time-Based Function-Call Generator/1
  connections:
  FIFO Queue/LConn1 -- Input/RConn1
  Release Gate/RConn1 -- Output/RConn1
  FIFO Queue/RConn1 -- Release Gate/LConn1

== system simple_router/Router12/Clocked FIFO2 ==
  Event-Based Random Number : EventBasedRandomNumber  Distribution=Gaussian (normal)  meanNorm=E  stdNorm=S
  FIFO Queue : FIFOQueue  Capacity=F  StatNumberInBlock=on
      settings: OutputPortMap=o1
  Release Gate : ReleaseGate  OpenGateUpon=Function call from port fcn
  Time-Based Function-Call Generator : TimeBasedFunctionCallGenerator  EventGenerationMode=Period from port  Period=T
  Input : PMIOPort  Port=1  Side=Left
  Output : PMIOPort  Port=2  Side=Right
  #n : Outport
  wires:
  Time-Based Function-Call Generator/1 -> Release Gate/1
  FIFO Queue/1 -> #n/1
  Event-Based Random Number/1 -> Time-Based Function-Call Generator/1
  connections:
  FIFO Queue/LConn1 -- Input/RConn1
  Release Gate/RConn1 -- Output/RConn1
  FIFO Queue/RConn1 -- Release Gate/LConn1

== system simple_router/Router12/Clocked FIFO3 ==
  Event-Based Random Number : EventBasedRandomNumber  Distribution=Gaussian (normal)  meanNorm=E  stdNorm=S
  FIFO Queue : FIFOQueue  Capacity=F  StatNumberInBlock=on
      settings: OutputPortMap=o1
  Release Gate : ReleaseGate  OpenGateUpon=Function call from port fcn
  Time-Based Function-Call Generator : TimeBasedFunctionCallGenerator  EventGenerationMode=Period from port  Period=T
  Input : PMIOPort  Port=1  Side=Left
  Output : PMIOPort  Port=2  Side=Right
  #n : Outport
  wires:
  Time-Based Function-Call Generator/1 -> Release Gate/1
  FIFO Queue/1 -> #n/1
  Event-Based Random Number/1 -> Time-Based Function-Call Generator/1
  connections:
  FIFO Queue/LConn1 -- Input/RConn1
  Release Gate/RConn1 -- Output/RConn1
  FIFO Queue/RConn1 -- Release Gate/LConn1

== system simple_router/Router12/Clocked FIFO4 ==
  Event-Based Random Number : EventBasedRandomNumber  Distribution=Gaussian (normal)  meanNorm=E  stdNorm=S
  FIFO Queue : FIFOQueue  Capacity=F  StatNumberInBlock=on
      settings: OutputPortMap=o1
  Release Gate : ReleaseGate  OpenGateUpon=Function call from port fcn
  Time-Based Function-Call Generator : TimeBasedFunctionCallGenerator  EventGenerationMode=Period from port  Period=T
  Input : PMIOPort  Port=1  Side=Left
  Output : PMIOPort  Port=2  Side=Right
  #n : Outport
  wires:
  Time-Based Function-Call Generator/1 -> Release Gate/1
  FIFO Queue/1 -> #n/1
  Event-Based Random Number/1 -> Time-Based Function-Call Generator/1
  connections:
  FIFO Queue/LConn1 -- Input/RConn1
  Release Gate/RConn1 -- Output/RConn1
  FIFO Queue/RConn1 -- Release Gate/LConn1

== system simple_router/Router12/Clocked FIFO5 ==
  Event-Based Random Number : EventBasedRandomNumber  Distribution=Gaussian (normal)  meanNorm=E  stdNorm=S
  FIFO Queue : FIFOQueue  Capacity=F  StatNumberInBlock=on
      settings: OutputPortMap=o1
  Release Gate : ReleaseGate  OpenGateUpon=Function call from port fcn
  Time-Based Function-Call Generator : TimeBasedFunctionCallGenerator  EventGenerationMode=Period from port  Period=T
  Input : PMIOPort  Port=1  Side=Left
  Output : PMIOPort  Port=2  Side=Right
  #n : Outport
  wires:
  Time-Based Function-Call Generator/1 -> Release Gate/1
  FIFO Queue/1 -> #n/1
  Event-Based Random Number/1 -> Time-Based Function-Call Generator/1
  connections:
  FIFO Queue/LConn1 -- Input/RConn1
  Release Gate/RConn1 -- Output/RConn1
  FIFO Queue/RConn1 -- Release Gate/LConn1

== system simple_router/Router13/Attribute Function ==
  MATLAB Function : MATLAB Function  TreatAsAtomicUnit=on
  __DMLF__EDE2FCE__ : EntityDepartureFunctionCallGenerator  TimingFunctionCallF1=Before entity departure  IsInsideAFB=on
  __DMLF__GA__ : GetAttribute  AttributeName=DST|ME  AttributeMissing=Error|Error  AttributeDefaultValue=1|1  AttributeTreatAsVector=1|1  AttributeSendTiming=Before entity departure|Before entity departure  EvaluatedDefaultAttributeValue={ [];[]}  IsInsideAFB=on
      settings: OutputPortMap=o1,o2
  __DMLF__SA__ : SetAttribute  AttributeName=RT  AttributeFrom=Signal port  EvaluatedAttributeValue={ []}  IsInsideAFB=on
  IN : PMIOPort  Port=1  Side=Left
  OUT : PMIOPort  Port=2  Side=Right
  wires:
  __DMLF__EDE2FCE__/1 -> MATLAB Function/Trigger
  __DMLF__GA__/1 -> MATLAB Function/1(DST)
  __DMLF__GA__/2 -> MATLAB Function/2(ME)
  MATLAB Function/1(out_RT) -> __DMLF__SA__/1
  connections:
  __DMLF__SA__/LConn1 -- __DMLF__EDE2FCE__/RConn1
  __DMLF__GA__/RConn1 -- __DMLF__EDE2FCE__/LConn1
  IN/RConn1 -- __DMLF__GA__/LConn1
  __DMLF__SA__/RConn1 -- OUT/RConn1

== system simple_router/Router13/Clocked FIFO1 ==
  Event-Based Random Number : EventBasedRandomNumber  Distribution=Gaussian (normal)  meanNorm=E  stdNorm=S
  FIFO Queue : FIFOQueue  Capacity=F  StatNumberInBlock=on
      settings: OutputPortMap=o1
  Release Gate : ReleaseGate  OpenGateUpon=Function call from port fcn
  Time-Based Function-Call Generator : TimeBasedFunctionCallGenerator  EventGenerationMode=Period from port  Period=T
  Input : PMIOPort  Port=1  Side=Left
  Output : PMIOPort  Port=2  Side=Right
  #n : Outport
  wires:
  Time-Based Function-Call Generator/1 -> Release Gate/1
  FIFO Queue/1 -> #n/1
  Event-Based Random Number/1 -> Time-Based Function-Call Generator/1
  connections:
  FIFO Queue/LConn1 -- Input/RConn1
  Release Gate/RConn1 -- Output/RConn1
  FIFO Queue/RConn1 -- Release Gate/LConn1

== system simple_router/Router13/Clocked FIFO2 ==
  Event-Based Random Number : EventBasedRandomNumber  Distribution=Gaussian (normal)  meanNorm=E  stdNorm=S
  FIFO Queue : FIFOQueue  Capacity=F  StatNumberInBlock=on
      settings: OutputPortMap=o1
  Release Gate : ReleaseGate  OpenGateUpon=Function call from port fcn
  Time-Based Function-Call Generator : TimeBasedFunctionCallGenerator  EventGenerationMode=Period from port  Period=T
  Input : PMIOPort  Port=1  Side=Left
  Output : PMIOPort  Port=2  Side=Right
  #n : Outport
  wires:
  Time-Based Function-Call Generator/1 -> Release Gate/1
  FIFO Queue/1 -> #n/1
  Event-Based Random Number/1 -> Time-Based Function-Call Generator/1
  connections:
  FIFO Queue/LConn1 -- Input/RConn1
  Release Gate/RConn1 -- Output/RConn1
  FIFO Queue/RConn1 -- Release Gate/LConn1

== system simple_router/Router13/Clocked FIFO3 ==
  Event-Based Random Number : EventBasedRandomNumber  Distribution=Gaussian (normal)  meanNorm=E  stdNorm=S
  FIFO Queue : FIFOQueue  Capacity=F  StatNumberInBlock=on
      settings: OutputPortMap=o1
  Release Gate : ReleaseGate  OpenGateUpon=Function call from port fcn
  Time-Based Function-Call Generator : TimeBasedFunctionCallGenerator  EventGenerationMode=Period from port  Period=T
  Input : PMIOPort  Port=1  Side=Left
  Output : PMIOPort  Port=2  Side=Right
  #n : Outport
  wires:
  Time-Based Function-Call Generator/1 -> Release Gate/1
  FIFO Queue/1 -> #n/1
  Event-Based Random Number/1 -> Time-Based Function-Call Generator/1
  connections:
  FIFO Queue/LConn1 -- Input/RConn1
  Release Gate/RConn1 -- Output/RConn1
  FIFO Queue/RConn1 -- Release Gate/LConn1

== system simple_router/Router13/Clocked FIFO4 ==
  Event-Based Random Number : EventBasedRandomNumber  Distribution=Gaussian (normal)  meanNorm=E  stdNorm=S
  FIFO Queue : FIFOQueue  Capacity=F  StatNumberInBlock=on
      settings: OutputPortMap=o1
  Release Gate : ReleaseGate  OpenGateUpon=Function call from port fcn
  Time-Based Function-Call Generator : TimeBasedFunctionCallGenerator  EventGenerationMode=Period from port  Period=T
  Input : PMIOPort  Port=1  Side=Left
  Output : PMIOPort  Port=2  Side=Right
  #n : Outport
  wires:
  Time-Based Function-Call Generator/1 -> Release Gate/1
  FIFO Queue/1 -> #n/1
  Event-Based Random Number/1 -> Time-Based Function-Call Generator/1
  connections:
  FIFO Queue/LConn1 -- Input/RConn1
  Release Gate/RConn1 -- Output/RConn1
  FIFO Queue/RConn1 -- Release Gate/LConn1
